simulink model "SIM_nonlinear"  (R2016a)
settings: Solver=ode23t  SolverMode=SingleTasking  StartTime=0.0  StopTime=20  MaxStep=1e-4  RelTol=1e-3
settings Model: Creator=edzel  LastModifiedBy=edzel
settings DataIOCC: ReturnWorkspaceOutputs=on
settings DebuggingCC: UnconnectedInputMsg=none  UnconnectedOutputMsg=none  UnconnectedLineMsg=none  SFUnexpectedBacktrackingDiag=error  SFNoUnconditionalDefaultTransitionDiag=error
settings ModelReferenceCC: EnableRefExpFcnMdlSchedulingChecks=off
settings SFSimCC: SimUseLocalCustomCode=on
settings RTWCC: Description=Generic Real-Time Target  RTWUseLocalCustomCode=on
settings GRTTargetCC: TargetLangStandard=C99 (ISO)
settings ConfigComp: CovMetricSettings=dwe  CovSaveCumulativeToWorkspaceVar=off  CovSaveSingleToWorkspaceVar=off  CovExternalEMLEnable=on

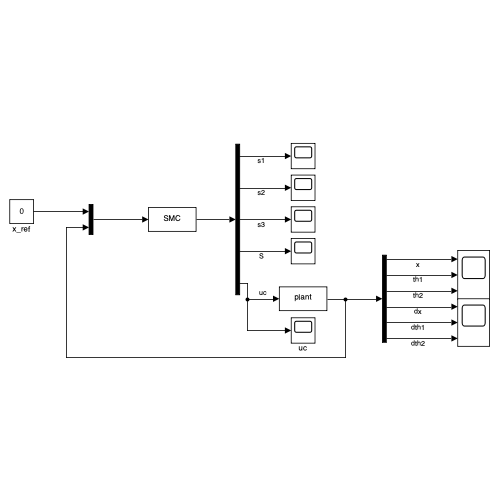
[thumbnail: Simulink's stored preview of the top-level diagram]
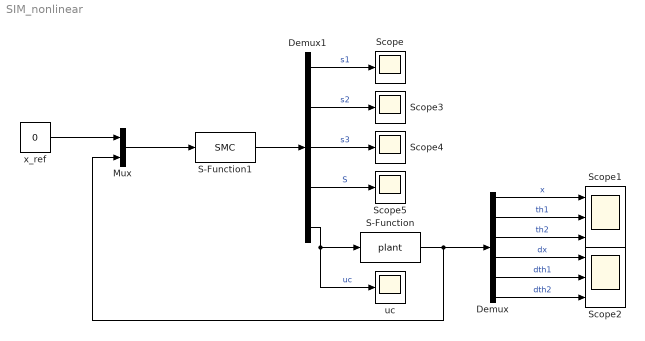
== system SIM_nonlinear ==
  Demux : Demux  Outputs=6
  Demux1 : Demux  Outputs=5
  Mux : Mux  Inputs=2
  S-Function : S-Function  FunctionName=plant  Parameters=CoeF1, CoeF2, CoeF3, theta1_rad, theta2_rad  SFunctionDeploymentMode=off  EnableBusSupport=off
  S-Function1 : S-Function  FunctionName=SMC  Parameters=CoeF1, CoeF2, CoeF3, para  SFunctionDeploymentMode=off  EnableBusSupport=off
  Scope{,3..5} (4 alike) : Scope
  Scope1 : Scope  NumInputPorts=3
  Scope2 : Scope  NumInputPorts=3
  uc : Scope
  x_ref : Constant  Value=0
  wires:
  x_ref/1 -> Mux/1
  Mux/1 -> S-Function1/1
  S-Function/1 -> Demux/1, Mux/2
  Demux/5 -> Scope2/2  "dth1"
  Demux/3 -> Scope1/3  "th2"
  Demux/1 -> Scope1/1  "x"
  Demux/2 -> Scope1/2  "th1"
  Demux/4 -> Scope2/1  "dx"
  Demux/6 -> Scope2/3  "dth2"
  Demux1/5 -> S-Function/1, uc/1  "uc"
  S-Function1/1 -> Demux1/1
  Demux1/1 -> Scope/1  "s1"
  Demux1/2 -> Scope3/1  "s2"
  Demux1/3 -> Scope4/1  "s3"
  Demux1/4 -> Scope5/1  "S"
